simulink subsystem "JD_from_datetime"  (R2022a)
settings: Solver=VariableStepAuto  StartTime=0.0  StopTime=10.0  RelTol=1e-3
settings Model: Creator=samuel  LastModifiedBy=samuel

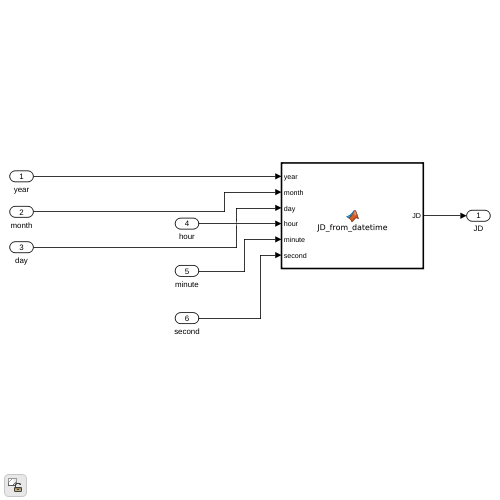
[thumbnail: Simulink's stored preview of the top-level diagram]
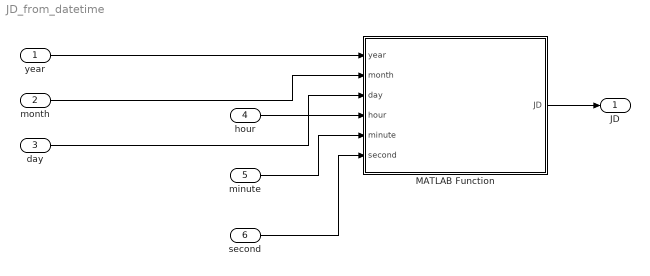
== system JD_from_datetime ==
  year : Inport
  month : Inport  Port=2
  day : Inport  Port=3
  hour : Inport  Port=4
  minute : Inport  Port=5
  second : Inport  Port=6
  MATLAB Function : MATLAB Function  TreatAsAtomicUnit=on
  JD : Outport
  wires:
  MATLAB Function/1(JD) -> JD/1
  day/1 -> MATLAB Function/3(day)
  second/1 -> MATLAB Function/6(second)
  hour/1 -> MATLAB Function/4(hour)
  year/1 -> MATLAB Function/1(year)
  minute/1 -> MATLAB Function/5(minute)
  month/1 -> MATLAB Function/2(month)

== matlab function JD_from_datetime/MATLAB Function ==
  data: year input; JD output; month input; day input; hour input; minute input; second input
function JD  = JD_from_datetime(year, month, day, hour, minute, second)

% Calculates the Julian date (JD) from the provided date (which must be
% between 1901 and 2099 for this calculation). Note that for days with a
% leap second, second / 61 should be used and this may need to be
% implemented in the future. For T0 calculations, seconds are 0 so this
% effect can be negelcted for this use case.

JD = 1721013.5 + 367*year - fix(7/4*(4+fix((month+9)/12))) + ...
    fix(275*month/9) + day + (60*hour + minute + second / 60) / 1440;
